simulink model "example_of_triggerd_subsystem"  (R2021a)
settings: Solver=FixedStepAuto  StartTime=0.0  StopTime=10  FixedStep=1e-3  RelTol=1e-3
settings Model: Creator=YasserNet  LastModifiedBy=YasserNet

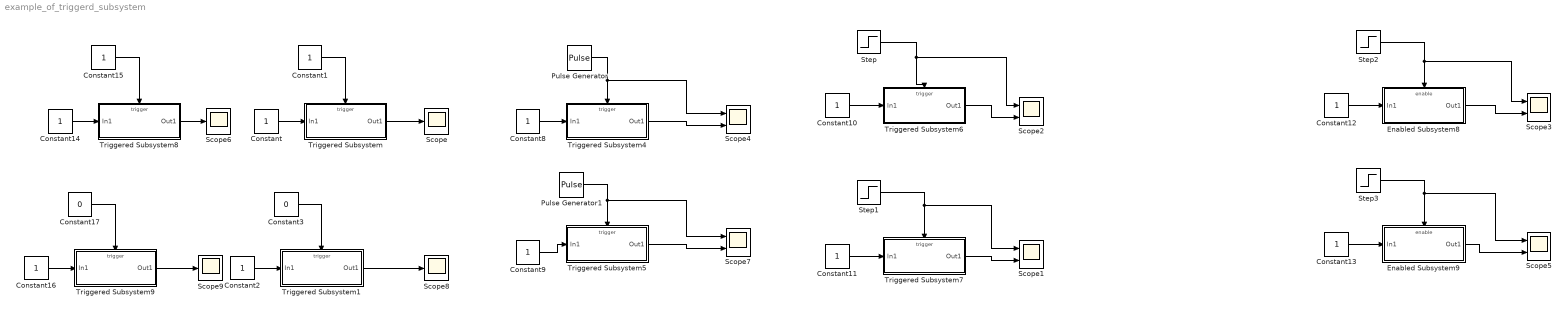
== system example_of_triggerd_subsystem ==
  Constant{,1..2,8..16} (12 alike) : Constant
  Constant17 : Constant  Value=0
  Constant3 : Constant  Value=0
  Enabled Subsystem8 : Subsystem  TreatAsAtomicUnit=on
  Enabled Subsystem9 : Subsystem  TreatAsAtomicUnit=on
  Pulse Generator : DiscretePulseGenerator  PulseType=Time based  PulseWidth=50
  Pulse Generator1 : DiscretePulseGenerator  PulseType=Time based  PulseWidth=50
  Scope{,6,8..9} (4 alike) : Scope
  Scope{1..5,7} (6 alike) : Scope  NumInputPorts=2
  Step : Step  SampleTime=0
  Step1 : Step  SampleTime=0
  Step2 : Step  Time=0  Before=-1  After=0  SampleTime=0
  Step3 : Step  Time=0  Before=1  After=2  SampleTime=0
  Triggered Subsystem : Subsystem  TreatAsAtomicUnit=on
  Triggered Subsystem1 : Subsystem  TreatAsAtomicUnit=on
  Triggered Subsystem4 : Subsystem  TreatAsAtomicUnit=on
  Triggered Subsystem5 : Subsystem  TreatAsAtomicUnit=on
  Triggered Subsystem6 : Subsystem  TreatAsAtomicUnit=on
  Triggered Subsystem7 : Subsystem  TreatAsAtomicUnit=on
  Triggered Subsystem8 : Subsystem  TreatAsAtomicUnit=on
  Triggered Subsystem9 : Subsystem  TreatAsAtomicUnit=on
  wires:
  Step/1 -> Scope2/1, Triggered Subsystem6/Trigger
  Step3/1 -> Scope5/1, Enabled Subsystem9/Enable
  Enabled Subsystem9/1(Out1) -> Scope5/2
  Pulse Generator1/1 -> Scope7/1, Triggered Subsystem5/Trigger
  Constant9/1 -> Triggered Subsystem5/1(In1)
  Triggered Subsystem1/1(Out1) -> Scope8/1
  Pulse Generator/1 -> Scope4/1, Triggered Subsystem4/Trigger
  Constant/1 -> Triggered Subsystem/1(In1)
  Triggered Subsystem6/1(Out1) -> Scope2/2
  Step1/1 -> Scope1/1, Triggered Subsystem7/Trigger
  Constant11/1 -> Triggered Subsystem7/1(In1)
  Constant10/1 -> Triggered Subsystem6/1(In1)
  Constant3/1 -> Triggered Subsystem1/Trigger
  Constant12/1 -> Enabled Subsystem8/1(In1)
  Enabled Subsystem8/1(Out1) -> Scope3/2
  Step2/1 -> Scope3/1, Enabled Subsystem8/Enable
  Triggered Subsystem5/1(Out1) -> Scope7/2
  Triggered Subsystem4/1(Out1) -> Scope4/2
  Constant8/1 -> Triggered Subsystem4/1(In1)
  Constant13/1 -> Enabled Subsystem9/1(In1)
  Triggered Subsystem/1(Out1) -> Scope/1
  Constant1/1 -> Triggered Subsystem/Trigger
  Constant2/1 -> Triggered Subsystem1/1(In1)
  Constant16/1 -> Triggered Subsystem9/1(In1)
  Constant15/1 -> Triggered Subsystem8/Trigger
  Triggered Subsystem8/1(Out1) -> Scope6/1
  Constant17/1 -> Triggered Subsystem9/Trigger
  Constant14/1 -> Triggered Subsystem8/1(In1)
  Triggered Subsystem9/1(Out1) -> Scope9/1
  Triggered Subsystem7/1(Out1) -> Scope1/2

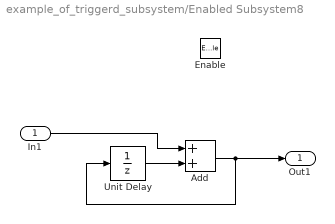
== system example_of_triggerd_subsystem/Enabled Subsystem8 ==
  In1 : Inport
  Enable : EnablePort
  Add : Sum
  Unit Delay : UnitDelay  HasFrameUpgradeWarning=on
  Out1 : Outport
  wires:
  Unit Delay/1 -> Add/2
  Add/1 -> Unit Delay/1, Out1/1
  In1/1 -> Add/1

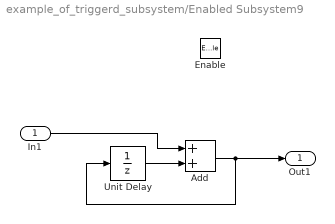
== system example_of_triggerd_subsystem/Enabled Subsystem9 ==
  In1 : Inport
  Enable : EnablePort
  Add : Sum
  Unit Delay : UnitDelay  HasFrameUpgradeWarning=on
  Out1 : Outport
  wires:
  In1/1 -> Add/1
  Add/1 -> Out1/1, Unit Delay/1
  Unit Delay/1 -> Add/2

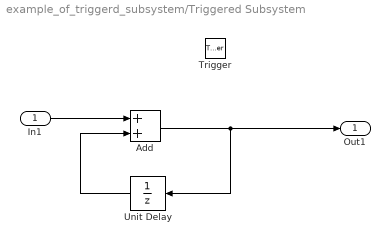
== system example_of_triggerd_subsystem/Triggered Subsystem ==
  In1 : Inport
  Trigger : TriggerPort  VariantControl=(inherit)
  Add : Sum
  Unit Delay : UnitDelay  SampleTime=-1  HasFrameUpgradeWarning=on
  Out1 : Outport
  wires:
  Add/1 -> Unit Delay/1, Out1/1
  In1/1 -> Add/1
  Unit Delay/1 -> Add/2

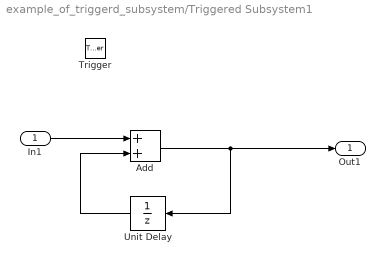
== system example_of_triggerd_subsystem/Triggered Subsystem1 ==
  In1 : Inport
  Trigger : TriggerPort  VariantControl=(inherit)
  Add : Sum
  Unit Delay : UnitDelay  SampleTime=-1  HasFrameUpgradeWarning=on
  Out1 : Outport
  wires:
  Unit Delay/1 -> Add/2
  In1/1 -> Add/1
  Add/1 -> Out1/1, Unit Delay/1

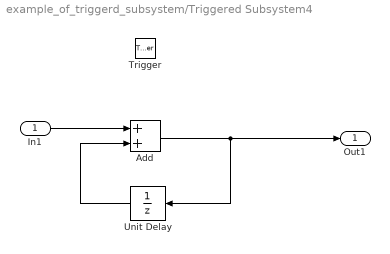
== system example_of_triggerd_subsystem/Triggered Subsystem4 ==
  In1 : Inport
  Trigger : TriggerPort  VariantControl=(inherit)
  Add : Sum
  Unit Delay : UnitDelay  SampleTime=-1  HasFrameUpgradeWarning=on
  Out1 : Outport
  wires:
  Unit Delay/1 -> Add/2
  In1/1 -> Add/1
  Add/1 -> Out1/1, Unit Delay/1

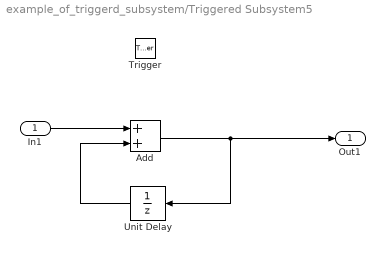
== system example_of_triggerd_subsystem/Triggered Subsystem5 ==
  In1 : Inport
  Trigger : TriggerPort  VariantControl=(inherit)
  Add : Sum
  Unit Delay : UnitDelay  SampleTime=-1  HasFrameUpgradeWarning=on
  Out1 : Outport
  wires:
  Unit Delay/1 -> Add/2
  In1/1 -> Add/1
  Add/1 -> Out1/1, Unit Delay/1

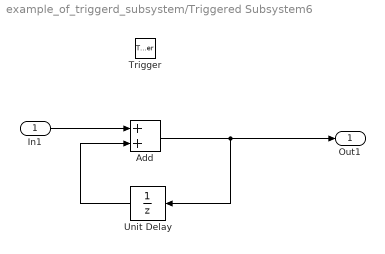
== system example_of_triggerd_subsystem/Triggered Subsystem6 ==
  In1 : Inport
  Trigger : TriggerPort  VariantControl=(inherit)
  Add : Sum
  Unit Delay : UnitDelay  SampleTime=-1  HasFrameUpgradeWarning=on
  Out1 : Outport
  wires:
  Unit Delay/1 -> Add/2
  In1/1 -> Add/1
  Add/1 -> Out1/1, Unit Delay/1

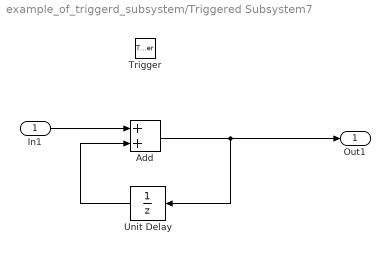
== system example_of_triggerd_subsystem/Triggered Subsystem7 ==
  In1 : Inport
  Trigger : TriggerPort  TriggerType=falling  VariantControl=(inherit)
  Add : Sum
  Unit Delay : UnitDelay  SampleTime=-1  HasFrameUpgradeWarning=on
  Out1 : Outport
  wires:
  Unit Delay/1 -> Add/2
  In1/1 -> Add/1
  Add/1 -> Out1/1, Unit Delay/1

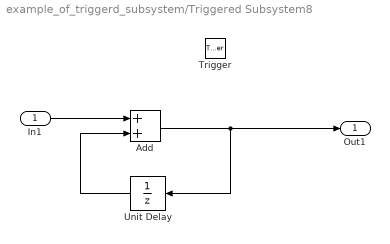
== system example_of_triggerd_subsystem/Triggered Subsystem8 ==
  In1 : Inport
  Trigger : TriggerPort  TriggerType=falling  VariantControl=(inherit)
  Add : Sum
  Unit Delay : UnitDelay  SampleTime=-1  HasFrameUpgradeWarning=on
  Out1 : Outport
  wires:
  Unit Delay/1 -> Add/2
  In1/1 -> Add/1
  Add/1 -> Out1/1, Unit Delay/1

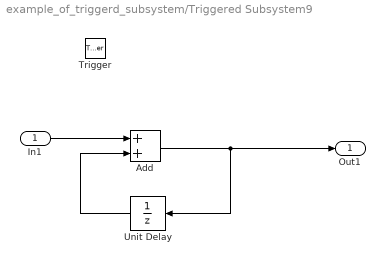
== system example_of_triggerd_subsystem/Triggered Subsystem9 ==
  In1 : Inport
  Trigger : TriggerPort  TriggerType=falling  VariantControl=(inherit)
  Add : Sum
  Unit Delay : UnitDelay  SampleTime=-1  HasFrameUpgradeWarning=on
  Out1 : Outport
  wires:
  Add/1 -> Unit Delay/1, Out1/1
  In1/1 -> Add/1
  Unit Delay/1 -> Add/2
